simulink model "miniProject2"  (Simulink 7.7)
settings: Solver=ode45  StartTime=0.0  StopTime=100  RelTol=1e-3
settings Model: Creator=jiannianweng  LastModifiedBy=jiannianweng

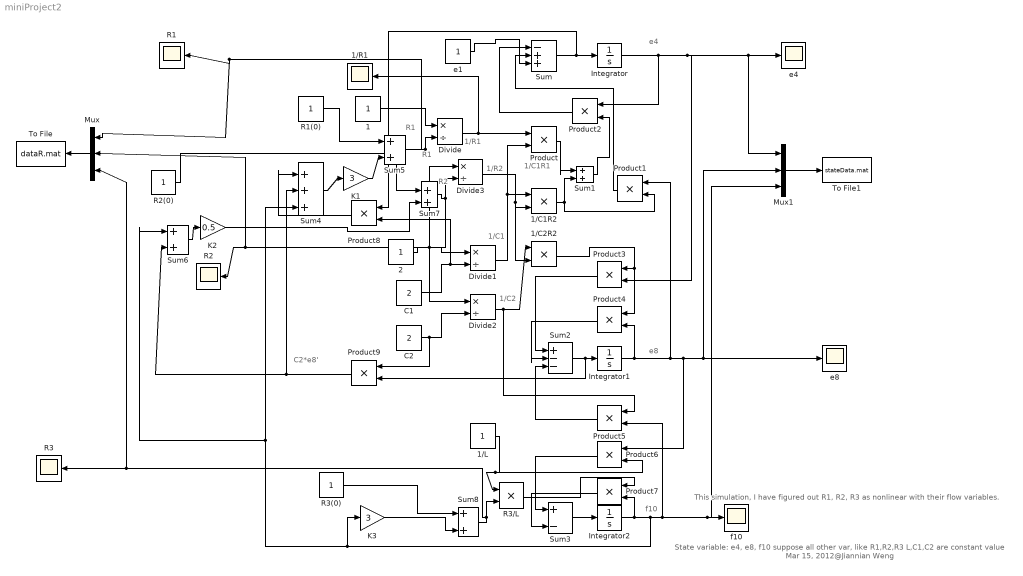
== system miniProject2 ==
  note: e4
  note: e8
  note: f10
  note: 1/C1R1
  note: State variable: e4, e8, f10
      | suppose all other var, like R1,R2,R3
      | L,C1,C2 are constant value
      | Mar 15, 2012@Jiannian Weng
  note: R1
  note: 1/R1
  note: This simulation, I have figured out R1, R2, R3 as nonlinear
      | with their flow variables.
  note: 1/C1
  note: 1/C2
  note: R1
  note: 1/R2
  note: C2*e8'
  note: R2
  1 : Constant
  1/C1R2 : Product  RndMeth=Zero
  1/C2R2 : Product  RndMeth=Zero
  1/L : Constant
  1/R1 : Scope
      settings: SaveName=ScopeData3
  2 : Constant
  C1 : Constant  Value=2
  C2 : Constant  Value=2
  Divide{,1..3} (4 alike) : Product  Inputs=*/
  Integrator : Integrator
  Integrator1 : Integrator
  Integrator2 : Integrator
  K1 : Gain  Gain=3
  K2 : Gain  Gain=0.5
  K3 : Gain  Gain=3
  Mux : Mux  Inputs=3
  Mux1 : Mux  Inputs=3
  Product{,1..9} (10 alike) : Product  RndMeth=Zero
  R1 : Scope
      settings: SaveName=ScopeData4
  R1(0) : Constant
  R2 : Scope
      settings: SaveName=ScopeData5
  R2(0) : Constant
  R3 : Scope
      settings: SaveName=ScopeData6
  R3(0) : Constant
  R3/L : Product  RndMeth=Zero
  Sum : Sum  Inputs=|-++
  Sum{1,5..8} (5 alike) : Sum  Inputs=|++
  Sum2 : Sum  Inputs=|+--
  Sum3 : Sum  Inputs=|+-
  Sum4 : Sum  Inputs=|+++
  To File : ToFile  Filename=dataR.mat  SaveFormat=Timeseries
  To File1 : ToFile  Filename=stateData.mat
  e1 : Constant
  e4 : Scope
  e8 : Scope
  f10 : Scope
      settings: SaveName=ScopeData2
  wires:
  Integrator/1 -> Product2/1, Product3/2, e4/1, Mux1/1
  Integrator1/1 -> Product1/1, Product6/1, e8/1, Mux1/2, Product4/2
  Integrator2/1 -> Product7/2, Product5/2, f10/1, Mux1/3, Sum4/3, Sum6/1, K3/1
  Sum/1 -> Integrator/1, Product8/1
  e1/1 -> Sum/3
  Divide1/1 -> Product/2, 1/C1R2/1
  Divide3/1 -> 1/C1R2/2, 1/C2R2/2
  Product/1 -> Sum1/1
  1/C1R2/1 -> Sum1/2, Product1/2
  Sum1/1 -> Product2/2
  Product2/1 -> Sum/1
  Product1/1 -> Sum/2
  Divide2/1 -> 1/C2R2/1, Product5/1
  1/C2R2/1 -> Product3/1, Product4/1
  Sum2/1 -> Integrator1/1, Product9/2
  Product3/1 -> Sum2/1
  Product4/1 -> Sum2/2
  Product5/1 -> Sum2/3
  Sum3/1 -> Integrator2/1
  1/L/1 -> Product6/2, R3/L/1
  Product6/1 -> Sum3/1
  Sum8/1 -> R3/L/2, R3/1, Mux/3
  R3/L/1 -> Product7/1
  Product7/1 -> Sum3/2
  Divide/1 -> Product/1, 1/R1/1
  1/1 -> Divide/1
  Sum5/1 -> Divide/2, R1/1, Mux/1
  2/1 -> Divide1/1, Divide2/1, Divide3/1
  C1/1 -> Divide1/2, Product8/2
  C2/1 -> Divide2/2, Product9/1
  Product8/1 -> Sum4/1
  Product9/1 -> Sum4/2, Sum6/2
  Sum4/1 -> K1/1
  R1(0)/1 -> Sum5/1
  K1/1 -> Sum5/2
  Sum6/1 -> K2/1
  Sum7/1 -> Divide3/2, R2/1, Mux/2
  R2(0)/1 -> Sum7/1
  K2/1 -> Sum7/2
  K3/1 -> Sum8/2
  R3(0)/1 -> Sum8/1
  Mux/1 -> To File/1
  Mux1/1 -> To File1/1
